simulink model "SVPWMtrials"  (R2015b)
settings: Solver=VariableStepAuto  StartTime=0.0  StopTime=1  RelTol=1e-3
libraries: powerlib x25
(part 1 of 3)
settings Model: Creator=hakan  LastModifiedBy=hakan

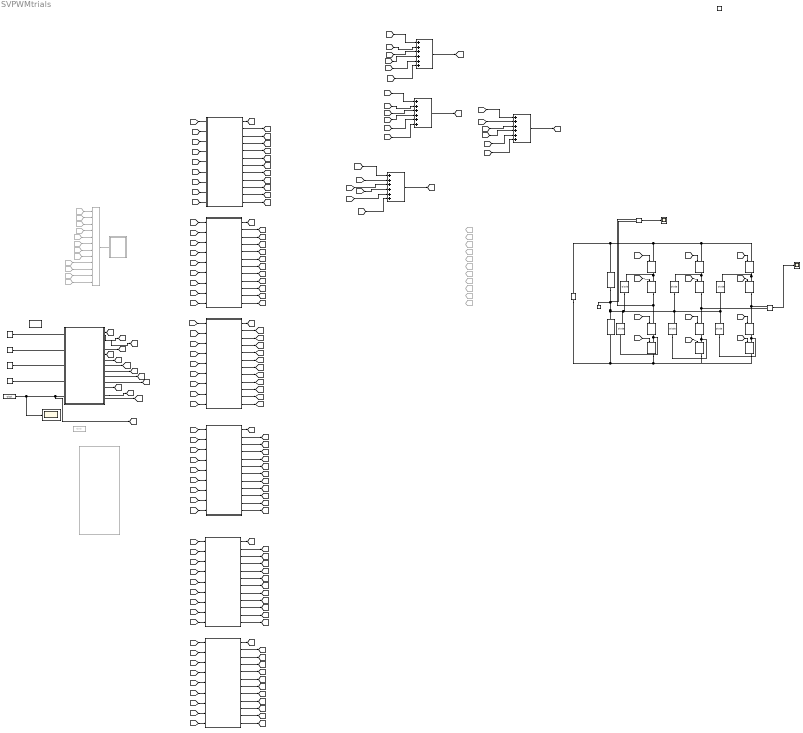
== system SVPWMtrials ==
  Enable : EnablePort
  Add{,1..3} (4 alike) : Sum  Inputs=++++++
  Bus Creator : BusCreator  Commented=on  Inputs=12
  Constant : Constant  Value=200
  Constant1 : Constant  Value=0.882
  Constant2 : Constant  Value=50
  Constant3 : Constant  Value=10000
  DC Voltage Source : powerlib/Electrical Sources/DC Voltage Source  Amplitude=100  Measurements=None
  Digital Clock : DigitalClock  SampleTime=0.000001
  Digital Clock1 : DigitalClock  Commented=on  SampleTime=0.000001
  Diode{1..6} (6 alike) : powerlib/Power Electronics/Diode  Ron=0.001  Lon=0  Vf=0.8  IC=0  UseSnubber=off  Rs=500  Cs=250e-9  Measurements=on
  From12 : From  Commented=on  GotoTag=Sa1
  From13 : From  Commented=on  GotoTag=Sa2
  From14 : From  Commented=on  GotoTag=Sa1P
  From15 : From  Commented=on  GotoTag=Sa2P
  From16 : From  Commented=on  GotoTag=Sb1
  From17 : From  Commented=on  GotoTag=Sb2
  From18 : From  Commented=on  GotoTag=Sb1P
  From19 : From  Commented=on  GotoTag=Sb2P
  From20 : From  Commented=on  GotoTag=Sc1
  From21 : From  Commented=on  GotoTag=Sc2
  From22 : From  Commented=on  GotoTag=Sc1P
  From23 : From  Commented=on  GotoTag=Sc2P
  Goto1 : Goto  Commented=on  GotoTag=Sa2
  Goto10 : Goto  Commented=on  GotoTag=Sc1P
  Goto11 : Goto  Commented=on  GotoTag=Sc2P
  Goto2 : Goto  Commented=on  GotoTag=Sa1P
  Goto3 : Goto  Commented=on  GotoTag=Sa2P
  Goto4 : Goto  Commented=on  GotoTag=Sb1
  Goto5 : Goto  Commented=on  GotoTag=Sb2
  Goto6 : Goto  Commented=on  GotoTag=Sb1P
  Goto7 : Goto  Commented=on  GotoTag=Sb2P
  Goto8 : Goto  Commented=on  GotoTag=Sc1
  Goto9 : Goto  Commented=on  GotoTag=Sc2
  Neutral : powerlib/Elements/Neutral  LConnTagsString=a  NodeNumber=10
  "Sa1 " : powerlib/Power Electronics/IGBT//Diode  Ron=1e-3  Rs=1e5  Cs=inf  Measurements=on
  Sa1P : powerlib/Power Electronics/IGBT//Diode  Ron=1e-3  Rs=1e5  Cs=inf  Measurements=on
  Sa2 : powerlib/Power Electronics/IGBT//Diode  Ron=1e-3  Rs=1e5  Cs=inf  Measurements=on
  Sa2P : powerlib/Power Electronics/IGBT//Diode  Ron=1e-3  Rs=1e5  Cs=inf  Measurements=on
  Sb1 : powerlib/Power Electronics/IGBT//Diode  Ron=1e-3  Rs=1e5  Cs=inf  Measurements=on
  Sb1P : powerlib/Power Electronics/IGBT//Diode  Ron=1e-3  Rs=1e5  Cs=inf  Measurements=on
  Sb2 : powerlib/Power Electronics/IGBT//Diode  Ron=1e-3  Rs=1e5  Cs=inf  Measurements=on
  Sb2P : powerlib/Power Electronics/IGBT//Diode  Ron=1e-3  Rs=1e5  Cs=inf  Measurements=on
  Sc1 : powerlib/Power Electronics/IGBT//Diode  Ron=1e-3  Rs=1e5  Cs=inf  Measurements=on
  Sc1P : powerlib/Power Electronics/IGBT//Diode  Ron=1e-3  Rs=1e5  Cs=inf  Measurements=on
  Sc2 : powerlib/Power Electronics/IGBT//Diode  Ron=1e-3  Rs=1e5  Cs=inf  Measurements=on
  Sc2P : powerlib/Power Electronics/IGBT//Diode  Ron=1e-3  Rs=1e5  Cs=inf  Measurements=on
  Scope : Scope
  Scope1 : Scope
  Scope2 : Scope
  Sector1 : MATLAB Function  TreatAsAtomicUnit=on
  Sector2 : MATLAB Function  TreatAsAtomicUnit=on
  Sector3 : MATLAB Function  TreatAsAtomicUnit=on
  Sector4 : MATLAB Function  TreatAsAtomicUnit=on
  Sector5 : MATLAB Function  TreatAsAtomicUnit=on
  Sector6 : MATLAB Function  TreatAsAtomicUnit=on
  Series RLC Branch : powerlib/Elements/Series RLC Branch  LConnTagsString=__new0  RConnTagsString=__new0  BranchType=RC  Resistance=1  Inductance=1e-3  SetiL0=off  InitialCurrent=0  Capacitance=1000e-6  Setx0=off  InitialVoltage=0  Measurements=None
  Series RLC Branch1 : powerlib/Elements/Series RLC Branch  LConnTagsString=__new0  RConnTagsString=__new0  BranchType=RC  Resistance=1  Inductance=1e-3  SetiL0=off  InitialCurrent=0  Capacitance=1000e-6  Setx0=off  InitialVoltage=0  Measurements=None
  Subsystem : Subsystem  Commented=on
  "Ta, Tb, Tc calc" : MATLAB Function  TreatAsAtomicUnit=on
  Voltage Measurement : powerlib/Measurements/Voltage Measurement  PhasorSimulation=off  OutputType=Complex  PSBequivalent=0
  Voltage Measurement1 : powerlib/Measurements/Voltage Measurement  PhasorSimulation=off  OutputType=Complex  PSBequivalent=0
  powergui : powerlib/powergui  Priority=1  SimulationMode=Continuous  SolverType=Tustin/Backward Euler (TBE)  SampleTime=50e-6  frequency=60  SPID=off  DisableSnubberDevices=off  DisableRonSwitches=off  DisableVfSwitches=off  SwTol=0  DisplayEquations=off  Interpol=off  ExternalGateDelay=off  methode=off  Ts=10  FunctionMessages=off  echomessages=off  HookPort=off  EnableUseOfTLC=off  x0status=blocks  frequencyindice=0  Pbase=100e6  ErrMax=1e-4  Iterations=50  UnitsV=kV  UnitsW=MW  buscounter=0  RestoreLinks=warning  ResistiveCurrentMeasurement=off  Frange=[0:2:500]  Ylog=off  Xlog=on  ShowGrid=off  save=off  variable=ZData  structure=dutycycles  ZoomFFT=off  StartTime=0.0  cycles=1  DisplayStyle=1  fundamental=5000  FreqAxis=off  MaxFrequency=10000  frequencyindicesteady=1  RmsSteady=1  display=off
  sequencing : MATLAB Function  Commented=on  TreatAsAtomicUnit=on
  wires:
  Constant/1 -> "Ta, Tb, Tc calc"/1(Vd)
  Constant1/1 -> "Ta, Tb, Tc calc"/2(ma)
  Constant2/1 -> "Ta, Tb, Tc calc"/3(fundf)
  Constant3/1 -> "Ta, Tb, Tc calc"/4(swf)
  Bus Creator/1 -> Subsystem/1(In1)
  [Sa1] -> "Sa1 "/1
  [Sa1P] -> Sa1P/1
  [Sa2] -> Sa2/1
  [Sa2P] -> Sa2P/1
  [Sb1] -> Sb1/1
  [Sb2] -> Sb2/1
  [Sb1P] -> Sb1P/1
  [Sb2P] -> Sb2P/1
  [Sc2P] -> Sc2P/1
  [Sc1P] -> Sc1P/1
  [Sc1] -> Sc1/1
  [Sc2] -> Sc2/1
  From12/1 -> Bus Creator/1
  From13/1 -> Bus Creator/2
  From14/1 -> Bus Creator/3
  From15/1 -> Bus Creator/4
  From16/1 -> Bus Creator/5
  From17/1 -> Bus Creator/6
  From18/1 -> Bus Creator/7
  From19/1 -> Bus Creator/8
  From20/1 -> Bus Creator/9
  From21/1 -> Bus Creator/10
  From22/1 -> Bus Creator/11
  From23/1 -> Bus Creator/12
  Voltage Measurement/1 -> Scope1/1
  Voltage Measurement1/1 -> Scope2/1
  Sector1/2(Sa2) -> [Sa21]
  Sector1/3(Sa1P) -> [Sa1P1]
  Sector1/4(Sa2P) -> [Sa2P1]
  Sector1/5(Sb1) -> [Sb11]
  Sector1/6(Sb2) -> [Sb21]
  Sector1/7(Sb1P) -> [Sb1P1]
  Sector1/8(Sb2P) -> [Sb2P1]
  Sector1/9(Sc1) -> [Sc11]
  Sector1/10(Sc2) -> [Sc21]
  Sector1/11(Sc1P) -> [Sc1P1]
  Sector1/12(Sc2P) -> [Sc2P1]
  Sector2/2(Sa2) -> [Sa22]
  Sector2/3(Sa1P) -> [Sa1P2]
  Sector2/4(Sa2P) -> [Sa2P2]
  Sector2/5(Sb1) -> [Sb12]
  Sector2/6(Sb2) -> [Sb22]
  Sector2/7(Sb1P) -> [Sb1P2]
  Sector2/8(Sb2P) -> [Sb2P2]
  Sector2/9(Sc1) -> [Sc12]
  Sector2/10(Sc2) -> [Sc22]
  Sector2/12(Sc2P) -> [Sc2P2]
  Sector2/11(Sc1P) -> [Sc1P2]
  "Ta, Tb, Tc calc"/1(rgn2a) -> [rgn2a]
  "Ta, Tb, Tc calc"/2(rgn2b) -> [rgn2b]
  "Ta, Tb, Tc calc"/3(rgn3) -> [rgn3]
  "Ta, Tb, Tc calc"/4(rgn4) -> [rgn4]
  "Ta, Tb, Tc calc"/12(Ta) -> [Ta]
  "Ta, Tb, Tc calc"/13(Tb) -> [Tb]
  "Ta, Tb, Tc calc"/14(Tc) -> [Tc]
  [Ta] -> Sector2/7(Ta)
  [Tb] -> Sector2/8(Tb)
  [Tc] -> Sector2/9(Tc)
  [rgn2a] -> Sector2/2(rgn2a)
  [rgn2b] -> Sector2/3(rgn2b)
  [rgn3] -> Sector2/4(rgn3)
  [rgn4] -> Sector2/5(rgn4)
  Digital Clock/1 -> [exttime], "Ta, Tb, Tc calc"/5(time), Scope/1
  [exttime] -> Sector2/6(exttime)
  [Tc] -> Sector3/9(Tc)
  [Tb] -> Sector3/8(Tb)
  [Ta] -> Sector3/7(Ta)
  [exttime] -> Sector3/6(exttime)
  [rgn4] -> Sector3/5(rgn4)
  [rgn3] -> Sector3/4(rgn3)
  [rgn2b] -> Sector3/3(rgn2b)
  [rgn2a] -> Sector3/2(rgn2a)
  [Tc] -> Sector4/9(Tc)
  [Tb] -> Sector4/8(Tb)
  [Ta] -> Sector4/7(Ta)
  [exttime] -> Sector4/6(exttime)
  [rgn4] -> Sector4/5(rgn4)
  [rgn3] -> Sector4/4(rgn3)
  [rgn2b] -> Sector4/3(rgn2b)
  [rgn2a] -> Sector4/2(rgn2a)
  [Tc] -> Sector5/9(Tc)
  [Tb] -> Sector5/8(Tb)
  [Ta] -> Sector5/7(Ta)
  [exttime] -> Sector5/6(exttime)
  [rgn4] -> Sector5/5(rgn4)
  [rgn3] -> Sector5/4(rgn3)
  [rgn2b] -> Sector5/3(rgn2b)
  [rgn2a] -> Sector5/2(rgn2a)
  [Tc] -> Sector6/9(Tc)
  [Tb] -> Sector6/8(Tb)
  [Ta] -> Sector6/7(Ta)
  [exttime] -> Sector6/6(exttime)
  [rgn4] -> Sector6/5(rgn4)
  [rgn3] -> Sector6/4(rgn3)
  [rgn2b] -> Sector6/3(rgn2b)
  [rgn2a] -> Sector6/2(rgn2a)
  [Ta] -> Sector1/7(Ta)
  [Tb] -> Sector1/8(Tb)
  [Tc] -> Sector1/9(Tc)
  [rgn2a] -> Sector1/2(rgn2a)
  [rgn2b] -> Sector1/3(rgn2b)
  [rgn3] -> Sector1/4(rgn3)
  [rgn4] -> Sector1/5(rgn4)
  [exttime] -> Sector1/6(exttime)
  "Ta, Tb, Tc calc"/6(Sector1) -> [Sector1]
  "Ta, Tb, Tc calc"/7(Sector2) -> [Sector2]
  "Ta, Tb, Tc calc"/8(Sector3) -> [Sector3]
  "Ta, Tb, Tc calc"/9(Sector4) -> [Sector4]
  "Ta, Tb, Tc calc"/10(Sector5) -> [Sector5]
  "Ta, Tb, Tc calc"/11(Sector6) -> [Sector6]
  [Sector1] -> Sector1/1(Sector1)
  [Sector2] -> Sector2/1(Sector2)
  [Sector3] -> Sector3/1(Sector3)
  [Sector4] -> Sector4/1(Sector4)
  [Sector5] -> Sector5/1(Sector5)
  [Sector6] -> Sector6/1(Sector6)
  Add/1 -> [Sa1]
  Sector1/1(Sa1) -> [Sa11]
  Sector2/1(Sa1) -> [Sa122]
  Sector3/1(Sa1) -> [Sa13]
  Sector4/1(Sa1) -> [Sa14]
  Sector5/1(Sa1) -> [Sa15]
  Sector6/1(Sa1) -> [Sa16]
  Sector3/12(Sc2P) -> [Sc2P3]
  Sector3/11(Sc1P) -> [Sc1P3]
  Sector3/10(Sc2) -> [Sc23]
  Sector3/9(Sc1) -> [Sc13]
  Sector3/8(Sb2P) -> [Sb2P3]
  Sector3/7(Sb1P) -> [Sb1P3]
  Sector3/6(Sb2) -> [Sb23]
  Sector3/5(Sb1) -> [Sb13]
  Sector3/4(Sa2P) -> [Sa2P3]
  Sector3/3(Sa1P) -> [Sa1P3]
  Sector3/2(Sa2) -> [Sa23]
  Sector4/2(Sa2) -> [Sa24]
  Sector4/3(Sa1P) -> [Sa1P4]
  Sector4/4(Sa2P) -> [Sa2P4]
  Sector4/5(Sb1) -> [Sb14]
  Sector4/6(Sb2) -> [Sb24]
  Sector4/7(Sb1P) -> [Sb1P4]
  Sector4/8(Sb2P) -> [Sb2P4]
  Sector4/9(Sc1) -> [Sc14]
  Sector4/10(Sc2) -> [Sc24]
  Sector4/11(Sc1P) -> [Sc1P4]
  Sector4/12(Sc2P) -> [Sc2P4]
  Sector5/2(Sa2) -> [Sa25]
  Sector5/3(Sa1P) -> [Sa1P5]
  Sector5/4(Sa2P) -> [Sa2P5]
  Sector5/5(Sb1) -> [Sb15]
  Sector5/6(Sb2) -> [Sb25]
  Sector5/7(Sb1P) -> [Sb1P5]
  Sector5/8(Sb2P) -> [Sb2P5]
  Sector5/9(Sc1) -> [Sc15]
  Sector5/10(Sc2) -> [Sc25]
  Sector5/11(Sc1P) -> [Sc1P5]
  Sector5/12(Sc2P) -> [Sc2P5]
  Sector6/12(Sc2P) -> [Sc2P6]
  Sector6/11(Sc1P) -> [Sc1P6]
  Sector6/10(Sc2) -> [Sc26]
  Sector6/9(Sc1) -> [Sc16]
  Sector6/8(Sb2P) -> [Sb2P6]
  Sector6/7(Sb1P) -> [Sb1P6]
  Sector6/6(Sb2) -> [Sb26]
  Sector6/5(Sb1) -> [Sb16]
  Sector6/4(Sa2P) -> [Sa2P6]
  Sector6/3(Sa1P) -> [Sa1P6]
  Sector6/2(Sa2) -> [Sa26]
  [Sa11] -> Add/1
  [Sa122] -> Add/2
  [Sa13] -> Add/3
  [Sa14] -> Add/4
  [Sa15] -> Add/5
  [Sa16] -> Add/6
  Add1/1 -> [Sa2]
  [Sa21] -> Add1/1
  [Sa22] -> Add1/2
  [Sa23] -> Add1/3
  [Sa24] -> Add1/4
  [Sa25] -> Add1/5
  [Sa26] -> Add1/6
  Add2/1 -> [Sa1P]
  [Sa1P1] -> Add2/1
  [Sa1P2] -> Add2/2
  [Sa1P3] -> Add2/3
  [Sa1P5] -> Add2/5
  [Sa1P6] -> Add2/6
  [Sa1P4] -> Add2/4
  Add3/1 -> [Sa2P]
  [Sa2P1] -> Add3/1
  [Sa2P3] -> Add3/3
  [Sa2P4] -> Add3/4
  [Sa2P5] -> Add3/5
  [Sa2P6] -> Add3/6
  [Sa2P2] -> Add3/2
  connections:
  DC Voltage Source/RConn1 -- Sc1/LConn1 -- Sb1/LConn1 -- "Sa1 "/LConn1 -- Series RLC Branch/LConn1
  DC Voltage Source/LConn1 -- Sb2P/RConn1 -- Sc2P/RConn1 -- Sa2P/RConn1 -- Series RLC Branch1/RConn1
  "Sa1 "/RConn1 -- Diode6/RConn1 -- Sa2/LConn1
  Sa2/RConn1 -- Voltage Measurement1/LConn1 -- Sa1P/LConn1
  Sa1P/RConn1 -- Diode1/LConn1 -- Sa2P/LConn1
  Sb1/RConn1 -- Diode3/RConn1 -- Sb2/LConn1
  Sb2/RConn1 -- Voltage Measurement/LConn2 -- Sb1P/LConn1
  Sb1P/RConn1 -- Diode2/LConn1 -- Sb2P/LConn1
  Sc1/RConn1 -- Diode4/RConn1 -- Sc2/LConn1
  Sc2/RConn1 -- Voltage Measurement/LConn1 -- Sc1P/LConn1
  Sc1P/RConn1 -- Diode5/LConn1 -- Sc2P/LConn1
  Diode6/LConn1 -- Voltage Measurement1/LConn2 -- Series RLC Branch/RConn1 -- Neutral/LConn1 -- Series RLC Branch1/LConn1 -- Diode3/LConn1 -- Diode5/RConn1 -- Diode4/LConn1 -- Diode2/RConn1 -- Diode1/RConn1

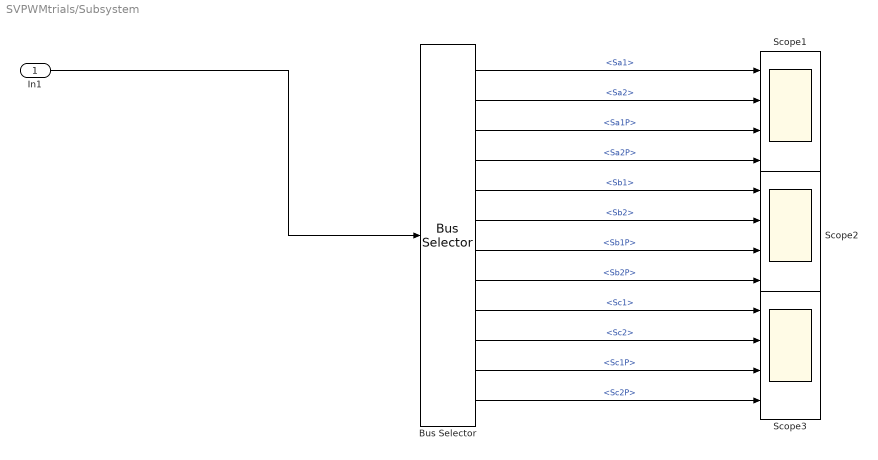
== system SVPWMtrials/Subsystem ==
  In1 : Inport
  Bus Selector : BusSelector  OutputSignals=Sa1,Sa2,Sa1P,Sa2P,Sb1,Sb2,Sb1P,Sb2P,Sc1,Sc2,Sc1P,Sc2P
  Scope1 : Scope  NumInputPorts=4
  Scope2 : Scope  NumInputPorts=4
  Scope3 : Scope  NumInputPorts=4
  wires:
  In1/1 -> Bus Selector/1
  Bus Selector/4 -> Scope1/4  "<Sa2P>"
  Bus Selector/3 -> Scope1/3  "<Sa1P>"
  Bus Selector/2 -> Scope1/2  "<Sa2>"
  Bus Selector/1 -> Scope1/1  "<Sa1>"
  Bus Selector/5 -> Scope2/1  "<Sb1>"
  Bus Selector/6 -> Scope2/2  "<Sb2>"
  Bus Selector/7 -> Scope2/3  "<Sb1P>"
  Bus Selector/8 -> Scope2/4  "<Sb2P>"
  Bus Selector/9 -> Scope3/1  "<Sc1>"
  Bus Selector/12 -> Scope3/4  "<Sc2P>"
  Bus Selector/11 -> Scope3/3  "<Sc1P>"
  Bus Selector/10 -> Scope3/2  "<Sc2>"

== matlab function SVPWMtrials/Ta, Tb, Tc calc ==
  data: rgn2a output; rgn2b output; rgn3 output; rgn4 output; angle output; Vd input; ma input; fundf input; swf input; time input; Sector1 output; Sector2 output; Sector3 output; Sector4 output; Sector5 output; Sector6 output; Ta output; Tb output; Tc output
function [rgn2a, rgn2b, rgn3, rgn4, angle, Sector1, Sector2, Sector3, Sector4, Sector5,Sector6, Ta, Tb, Tc] = fcn(Vd,ma,fundf, swf, time)
% this program works for magnitude of Vref is greater then Vd/3 meaning ma
% must be greater than 1/sqrt(3). for smaller ma's computation is a bit
% more tricky therefore it is omitted for simplicity for now. 
%#ok<*NASGU>
Vref = ma*Vd/sqrt(3); %magnitude of Vref
theta = 2*pi*fundf*time; %angle of Vref
angle = mod(theta, 2*pi);
Ts = 1/swf;
Ta = 0;
Tb = 0;
Tc = 0;
output = 0;
Sector1 = 0; Sector2 = 0; Sector3 = 0; Sector4= 0; Sector5 = 0; Sector6 = 0;
rgn2a = 0 ;rgn2b = 0; rgn3 = 0; rgn4 = 0;
Sa1=0; Sa2=0; Sa1P=0; Sa2P=0; Sb1=0; Sb2=0; Sb1P=0; Sb2P=0; Sc1=0; Sc2=0; Sc1P=0; Sc2P=0;
anglefrom3to2= 0 ;
%% Sector 1


if (mod(theta, 2*pi)<=pi/3)&&(mod(theta, 2*pi)>=0)  % sector 1

    n = 1;
    thetaprime = theta - (n-1)*pi/3;
        for aci = 0:0.00001:pi/3   
            la = sqrt(3)*cos(aci)-sin(aci);
                if (la*ma >= 0.99)&&(la*ma<=1)
                    anglefrom3to2 = aci; %leaving angle from region 3 to region 2
                    break
                end
        end

    %anglefrom3to2 = asin(1-1/(sqrt(3)*ma)); 
    anglefrom2to4 = pi/3 - anglefrom3to2; %leaving angle from region 2 to region 4
    if (mod(theta, 2*pi)<=anglefrom3to2) % then sector 1 region 3
        rgn2a = 0 ;rgn2b = 0; rgn3 = 1; rgn4 = 0;
        Ta = Ts*(2-2*ma*sin(pi/3+thetaprime));
        Tb = Ts*2*ma*sin(thetaprime);
        Tc = Ts*(2*ma*sin(pi/3-thetaprime)-1);        
    else if (mod(theta,2*pi)>=anglefrom3to2)&&(mod(theta,2*pi)<=anglefrom2to4) % then sector 1 region 2
            if angle<= pi/6 % then 2a
                rgn2a= 1; rgn2b = 0; rgn3 = 0; rgn4=0;
            else % then 2b
                rgn2a= 0; rgn2b = 1; rgn3 = 0; rgn4=0;
            end
            Ta = Ts*(1-2*ma*sin(thetaprime));
            Tb = Ts*(2*ma*sin(pi/3+thetaprime)-1);
            Tc = Ts*(1-2*ma*sin(pi/3-thetaprime));       
        else if (mod(theta,2*pi)>=anglefrom2to4) % then sector 1 region 4
               rgn2a = 0 ;rgn2b = 0; rgn3 = 0; rgn4 = 1;
               Ta = Ts*(2*ma*sin(thetaprime)-1);
               Tb = Ts*(2*ma*sin(pi/3-thetaprime));
               Tc = Ts*(2-2*ma*sin(pi/3+thetaprime));               
            end
        end
    end
    Sector1 = 1; Sector2 = 0; Sector3 = 0; Sector4= 0; Sector5 = 0; Sector6 = 0;
end
%% Sector 2


if (mod(theta, 2*pi)<=2*pi/3)&&(mod(theta, 2*pi)>=pi/3)  % sector 2
    
    n = 2;
    thetaprime = theta - (n-1)*pi/3;
        for aci = 0:0.00001:pi/3   
            la = sqrt(3)*cos(aci)-sin(aci);
                if (la*ma >= 0.99)&&(la*ma<=1)
                    anglefrom3to2 = aci; %leaving angle from region 3 to region 2
                    break
                end
        end
    %anglefrom3to2 = pi/3 + asin(1-1/(sqrt(3)*ma));
    anglefrom2to4 = pi/3 + pi/3 - anglefrom3to2;
    if (mod(theta, 2*pi)<=anglefrom3to2) % then sector 2 region 3
        rgn2a = 0 ;rgn2b = 0; rgn3 = 1; rgn4 = 0;
        Ta = Ts*(2-2*ma*sin(pi/3+thetaprime));
        Tb = Ts*2*ma*sin(thetaprime);
        Tc = Ts*(2*ma*sin(pi/3-thetaprime)-1); 
    else if (mod(theta,2*pi)>=anglefrom3to2)&&(mod(theta,2*pi)<=anglefrom2to4) % then sector 2 region 2
            if angle<=pi/2 %then 2a
                rgn2a= 1; rgn2b = 0; rgn3 = 0; rgn4=0;
            else % then 2b
                rgn2a= 0; rgn2b = 1; rgn3 = 0; rgn4=0;
            end
            Ta = Ts*(1-2*ma*sin(thetaprime));
            Tb = Ts*(2*ma*sin(pi/3+thetaprime)-1);
            Tc = Ts*(1-2*ma*sin(pi/3-thetaprime)); 
        else if (mod(theta,2*pi)>=anglefrom2to4) % then sector 2 region 4
               rgn2a = 0 ;rgn2b = 0; rgn3 = 0; rgn4 = 1;
               Ta = Ts*(2*ma*sin(thetaprime)-1);
               Tb = Ts*(2*ma*sin(pi/3-thetaprime));
               Tc = Ts*(2-2*ma*sin(pi/3+thetaprime)); 
            end
        end
    end
    Sector1 = 0; Sector2 = 1; Sector3 = 0; Sector4= 0; Sector5 = 0; Sector6 = 0;
end
%% Sector 3

if (mod(theta, 2*pi)<=pi)&&(mod(theta, 2*pi)>=2*pi/3)  % sector 3
    
    n = 3;
    thetaprime = theta - (n-1)*pi/3;
        for aci = 0:0.00001:pi/3   
            la = sqrt(3)*cos(aci)-sin(aci);
                if (la*ma >= 0.99)&&(la*ma<=1)
                    anglefrom3to2 = aci; %leaving angle from region 3 to region 2
                    break
                end
        end    
    %anglefrom3to2 = 2*pi/3 + asin(1-1/(sqrt(3)*ma));
    anglefrom2to4 = 2*pi/3 + pi/3 - anglefrom3to2;
    if (mod(theta, 2*pi)<=anglefrom3to2) % then sector 3 region 3
        rgn2a = 0 ;rgn2b = 0; rgn3 = 1; rgn4 = 0;
        Ta = Ts*(2-2*ma*sin(pi/3+thetaprime));
        Tb = Ts*2*ma*sin(thetaprime);
        Tc = Ts*(2*ma*sin(pi/3-thetaprime)-1); 
    else if (mod(theta,2*pi)>=anglefrom3to2)&&(mod(theta,2*pi)<=anglefrom2to4) % then sector 3 region 2
            if angle<=5*pi/6 %then 2a
                rgn2a= 1; rgn2b = 0; rgn3 = 0; rgn4=0;
            else % then 2b
                rgn2a= 0; rgn2b = 1; rgn3 = 0; rgn4=0;
            end
            Ta = Ts*(1-2*ma*sin(thetaprime));
            Tb = Ts*(2*ma*sin(pi/3+thetaprime)-1);
            Tc = Ts*(1-2*ma*sin(pi/3-thetaprime)); 
        else if (mod(theta,2*pi)>=anglefrom2to4) % then sector 3 region 4
                rgn2a = 0 ;rgn2b = 0; rgn3 = 0; rgn4 = 1;
               Ta = Ts*(2*ma*sin(thetaprime)-1);
               Tb = Ts*(2*ma*sin(pi/3-thetaprime));
               Tc = Ts*(2-2*ma*sin(pi/3+thetaprime)); 
            end
        end
    end
    Sector1 = 0; Sector2 = 0; Sector3 = 1; Sector4= 0; Sector5 = 0; Sector6 = 0;
end

%% Sector 4


if (mod(theta, 2*pi)<=4*pi/3)&&(mod(theta, 2*pi)>=pi)  % sector 4
    

    n = 4;
    thetaprime = theta - (n-1)*pi/3;
        for aci = 0:0.00001:pi/3   
            la = sqrt(3)*cos(aci)-sin(aci);
                if (la*ma >= 0.99)&&(la*ma<=1)
                    anglefrom3to2 = aci; %leaving angle from region 3 to region 2
                    break
                end
        end    
    %anglefrom3to2 = pi + asin(1-1/(sqrt(3)*ma));
    anglefrom2to4 = pi + pi/3 - anglefrom3to2;
    if (mod(theta, 2*pi)<=anglefrom3to2) % then sector 4 region 3
        rgn2a = 0 ;rgn2b = 0; rgn3 = 1; rgn4 = 0;
        Ta = Ts*(2-2*ma*sin(pi/3+thetaprime));
        Tb = Ts*2*ma*sin(thetaprime);
        Tc = Ts*(2*ma*sin(pi/3-thetaprime)-1); 
    else if (mod(theta,2*pi)>=anglefrom3to2)&&(mod(theta,2*pi)<=anglefrom2to4) % then sector 4 region 2
            if angle<=7*pi/6 %then 2a
                rgn2a= 1; rgn2b = 0; rgn3 = 0; rgn4=0;
            else % then 2b
                rgn2a= 0; rgn2b = 1; rgn3 = 0; rgn4=0;
            end
            Ta = Ts*(1-2*ma*sin(thetaprime));
            Tb = Ts*(2*ma*sin(pi/3+thetaprime)-1);
            Tc = Ts*(1-2*ma*sin(pi/3-thetaprime));
        else if (mod(theta,2*pi)>=anglefrom2to4) % then sector 4 region 4
                rgn2a = 0 ;rgn2b = 0; rgn3 = 0; rgn4 = 1;
               Ta = Ts*(2*ma*sin(thetaprime)-1);
               Tb = Ts*(2*ma*sin(pi/3-thetaprime));
               Tc = Ts*(2-2*ma*sin(pi/3+thetaprime)); 
            end
        end
    end
    Sector1 = 0; Sector2 = 0; Sector3 = 0; Sector4= 1; Sector5 = 0; Sector6 = 0;
end
%% Sector 5 

if (mod(theta, 2*pi)<=5*pi/3)&&(mod(theta, 2*pi)>=4*pi/3)  % sector 5
    
    n = 5;
    thetaprime = theta - (n-1)*pi/3;
    %anglefrom3to2 = 4*pi/3 + asin(1-1/(sqrt(3)*ma));
        for aci = 0:0.00001:pi/3   
            la = sqrt(3)*cos(aci)-sin(aci);
                if (la*ma >= 0.99)&&(la*ma<=1)
                    anglefrom3to2 = aci; %leaving angle from region 3 to region 2
                    break
                end
        end    
    anglefrom2to4 = 4*pi/3 + pi/3 - anglefrom3to2;
    if (mod(theta, 2*pi)<=anglefrom3to2) % then sector 5 region 3
        rgn2a = 0 ;rgn2b = 0; rgn3 = 1; rgn4 = 0;
        Ta = Ts*(2-2*ma*sin(pi/3+thetaprime));
        Tb = Ts*2*ma*sin(thetaprime);
        Tc = Ts*(2*ma*sin(pi/3-thetaprime)-1); 
    else if (mod(theta,2*pi)>=anglefrom3to2)&&(mod(theta,2*pi)<=anglefrom2to4) % then sector 5 region 2
            if angle<=3*pi/2 %then 2a
                rgn2a= 1; rgn2b = 0; rgn3 = 0; rgn4=0;
            else % then 2b
                rgn2a= 0; rgn2b = 1; rgn3 = 0; rgn4=0;
            end
            Ta = Ts*(1-2*ma*sin(thetaprime));
            Tb = Ts*(2*ma*sin(pi/3+thetaprime)-1);
            Tc = Ts*(1-2*ma*sin(pi/3-thetaprime));
        else if (mod(theta,2*pi)>=anglefrom2to4) % then sector 5 region 4
               rgn2a = 0 ;rgn2b = 0; rgn3 = 0; rgn4 = 1;
               Ta = Ts*(2*ma*sin(thetaprime)-1);
               Tb = Ts*(2*ma*sin(pi/3-thetaprime));
               Tc = Ts*(2-2*ma*sin(pi/3+thetaprime)); 
            end
        end
    end
    Sector1 = 0; Sector2 = 0; Sector3 = 0; Sector4= 0; Sector5 = 1; Sector6 = 0;
end

%% Sector 6 

if (mod(theta, 2*pi)<=2*pi)&&(mod(theta, 2*pi)>=5*pi/3)  % sector 6
    
    n = 6;
    thetaprime = theta - (n-1)*pi/3;
        for aci = 0:0.00001:pi/3   
            la = sqrt(3)*cos(aci)-sin(aci);
                if (la*ma >= 0.99)&&(la*ma<=1)
                    anglefrom3to2 = aci; %leaving angle from region 3 to region 2
                    break
                end
        end    
    %anglefrom3to2 = 5*pi/3 + asin(1-1/(sqrt(3)*ma));
    anglefrom2to4 = 5*pi/3 + pi/3 - anglefrom3to2;
    if (mod(theta, 2*pi)<=anglefrom3to2) % then sector 6 region 3
        rgn2a = 0 ;rgn2b = 0; rgn3 = 1; rgn4 = 0;
        Ta = Ts*(2-2*ma*sin(pi/3+thetaprime));
        Tb = Ts*2*ma*sin(thetaprime);
        Tc = Ts*(2*ma*sin(pi/3-thetaprime)-1); 
    else if (mod(theta,2*pi)>=anglefrom3to2)&&(mod(theta,2*pi)<=anglefrom2to4) % then sector 6 region 2
            if angle<=11*pi/6 %then 2a
                rgn2a= 1; rgn2b = 0; rgn3 = 0; rgn4=0;
            else % then 2b
                rgn2a= 0; rgn2b = 1; rgn3 = 0; rgn4=0;
            end
            Ta = Ts*(1-2*ma*sin(thetaprime));
            Tb = Ts*(2*ma*sin(pi/3+thetaprime)-1);
            Tc = Ts*(1-2*ma*sin(pi/3-thetaprime));
        else if (mod(theta,2*pi)>=anglefrom2to4) % then sector 6 region 4
               rgn2a = 0 ;rgn2b = 0; rgn3 = 0; rgn4 = 1;
               Ta = Ts*(2*ma*sin(thetaprime)-1);
               Tb = Ts*(2*ma*sin(pi/3-thetaprime));
               Tc = Ts*(2-2*ma*sin(pi/3+thetaprime)); 
            end
        end
    end
    Sector1 = 0; Sector2 = 0; Sector3 = 0; Sector4= 0; Sector5 = 0; Sector6 = 1;
end
